simulink model "Counters"  (R2022a)
settings: Solver=FixedStepAuto  StartTime=0.0  StopTime=10.0  FixedStep=0.5  RelTol=1e-3
settings Model: Creator=SALAH  LastModifiedBy=SALAH

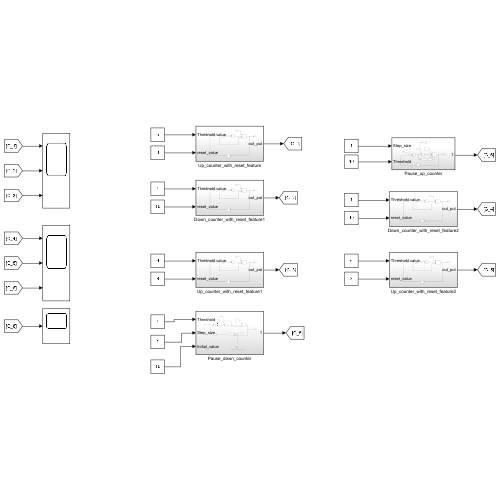
[thumbnail: Simulink's stored preview of the top-level diagram]
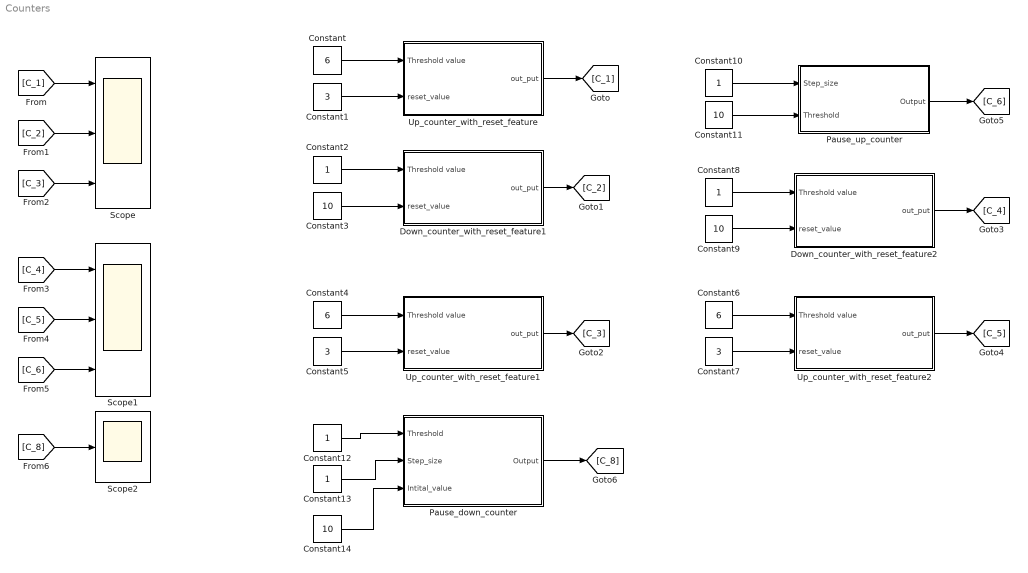
== system Counters ==
  Constant : Constant  Value=6
  Constant1 : Constant  Value=3
  Constant{2,8,10,12..13} (5 alike) : Constant
  Constant{3,9,11,14} (4 alike) : Constant  Value=10
  Constant4 : Constant  Value=6
  Constant5 : Constant  Value=3
  Constant6 : Constant  Value=6
  Constant7 : Constant  Value=3
  Down_counter_with_reset_feature1 : Subsystem
  Down_counter_with_reset_feature2 : Subsystem  Priority=2
  Pause_down_counter : Subsystem
  Pause_up_counter : Subsystem
  Scope : Scope  NumInputPorts=3
  Scope1 : Scope  NumInputPorts=3
  Scope2 : Scope
  Up_counter_with_reset_feature : Subsystem
  Up_counter_with_reset_feature1 : Subsystem
  Up_counter_with_reset_feature2 : Subsystem  Priority=1
  wires:
  Constant/1 -> Up_counter_with_reset_feature/1(Threshold value)
  Constant1/1 -> Up_counter_with_reset_feature/2(reset_value)
  Constant3/1 -> Down_counter_with_reset_feature1/2(reset_value)
  Constant2/1 -> Down_counter_with_reset_feature1/1(Threshold value)
  Constant5/1 -> Up_counter_with_reset_feature1/2(reset_value)
  Constant4/1 -> Up_counter_with_reset_feature1/1(Threshold value)
  Constant6/1 -> Up_counter_with_reset_feature2/1(Threshold value)
  Constant7/1 -> Up_counter_with_reset_feature2/2(reset_value)
  Up_counter_with_reset_feature/1(out_put) -> [C_1]
  Down_counter_with_reset_feature1/1(out_put) -> [C_2]
  Up_counter_with_reset_feature1/1(out_put) -> [C_3]
  Down_counter_with_reset_feature2/1(out_put) -> [C_4]
  Up_counter_with_reset_feature2/1(out_put) -> [C_5]
  [C_1] -> Scope/1
  [C_2] -> Scope/2
  [C_3] -> Scope/3
  [C_4] -> Scope1/1
  [C_5] -> Scope1/2
  Constant8/1 -> Down_counter_with_reset_feature2/1(Threshold value)
  Constant9/1 -> Down_counter_with_reset_feature2/2(reset_value)
  Constant10/1 -> Pause_up_counter/1(Step_size)
  Constant11/1 -> Pause_up_counter/2(Threshold)
  Pause_up_counter/1(Output) -> [C_6]
  [C_6] -> Scope1/3
  Constant12/1 -> Pause_down_counter/1(Threshold)
  Constant13/1 -> Pause_down_counter/2(Step_size)
  Pause_down_counter/1(Output) -> [C_8]
  [C_8] -> Scope2/1
  Constant14/1 -> Pause_down_counter/3(Intital_value)

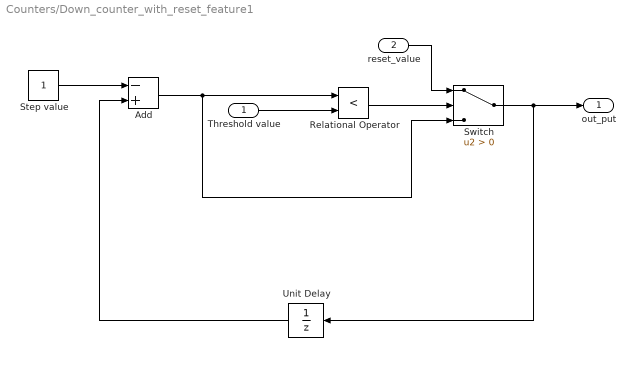
== system Counters/Down_counter_with_reset_feature1 ==
  Threshold value : Inport
  reset_value : Inport  Port=2
  Add : Sum  Inputs=-+
  Relational Operator : RelationalOperator  Operator=<  OutDataTypeStr=boolean  RndMeth=Simplest  InputSameDT=off
  Step value : Constant
  Switch : Switch  Criteria=u2 > Threshold  SaturateOnIntegerOverflow=off  InputSameDT=off
  Unit Delay : UnitDelay  SampleTime=-1  HasFrameUpgradeWarning=on
  out_put : Outport
  wires:
  reset_value/1 -> Switch/1
  Add/1 -> Relational Operator/1, Switch/3
  Unit Delay/1 -> Add/2
  Switch/1 -> Unit Delay/1, out_put/1
  Threshold value/1 -> Relational Operator/2
  Relational Operator/1 -> Switch/2
  Step value/1 -> Add/1

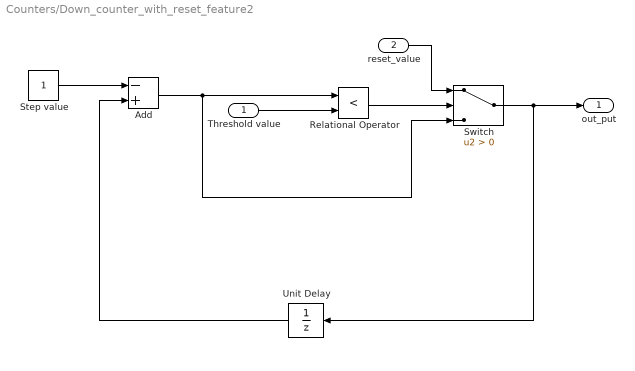
== system Counters/Down_counter_with_reset_feature2 ==
  Threshold value : Inport
  reset_value : Inport  Port=2
  Add : Sum  Inputs=-+
  Relational Operator : RelationalOperator  Operator=<  OutDataTypeStr=boolean  RndMeth=Simplest  InputSameDT=off
  Step value : Constant
  Switch : Switch  Criteria=u2 > Threshold  SaturateOnIntegerOverflow=off  InputSameDT=off
  Unit Delay : UnitDelay  SampleTime=-1  HasFrameUpgradeWarning=on
  out_put : Outport
  wires:
  Step value/1 -> Add/1
  Relational Operator/1 -> Switch/2
  Threshold value/1 -> Relational Operator/2
  Switch/1 -> out_put/1, Unit Delay/1
  Unit Delay/1 -> Add/2
  Add/1 -> Switch/3, Relational Operator/1
  reset_value/1 -> Switch/1

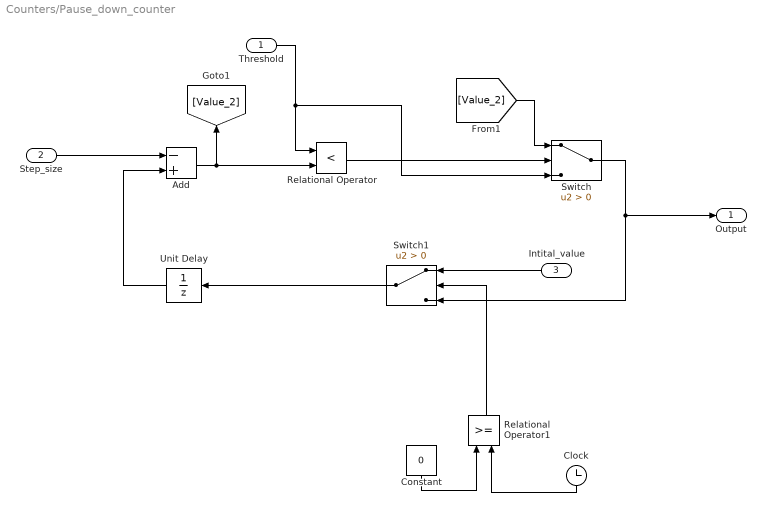
== system Counters/Pause_down_counter ==
  Threshold : Inport
  Step_size : Inport  Port=2
  Intital_value : Inport  Port=3
  Add : Sum  Inputs=-+
  Clock : Clock
  Constant : Constant  Value=0
  Relational Operator : RelationalOperator  Operator=<  OutDataTypeStr=boolean  RndMeth=Simplest  InputSameDT=off
  Relational Operator1 : RelationalOperator  Priority=1  OutDataTypeStr=boolean  RndMeth=Simplest  InputSameDT=off
  Switch : Switch  Criteria=u2 > Threshold  SaturateOnIntegerOverflow=off  InputSameDT=off
  Switch1 : Switch  Priority=2  Criteria=u2 > Threshold  SaturateOnIntegerOverflow=off  InputSameDT=off
  Unit Delay : UnitDelay  Priority=3  SampleTime=-1  HasFrameUpgradeWarning=on
  Output : Outport
  wires:
  Add/1 -> Relational Operator/2, [Value_2]
  Unit Delay/1 -> Add/2
  Relational Operator/1 -> Switch/2
  Threshold/1 -> Switch/3, Relational Operator/1
  Step_size/1 -> Add/1
  [Value_2] -> Switch/1
  Clock/1 -> Relational Operator1/2
  Constant/1 -> Relational Operator1/1
  Switch1/1 -> Unit Delay/1
  Switch/1 -> Switch1/3, Output/1
  Relational Operator1/1 -> Switch1/2
  Intital_value/1 -> Switch1/1

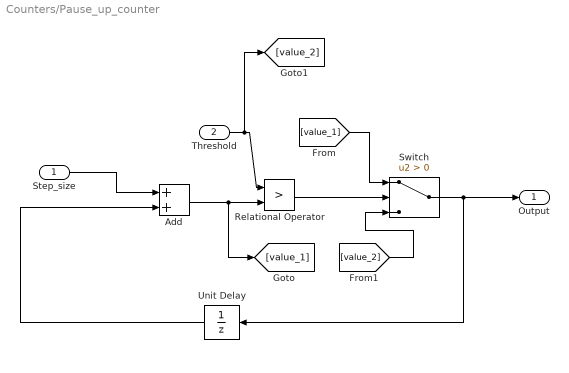
== system Counters/Pause_up_counter ==
  Step_size : Inport
  Threshold : Inport  Port=2
  Add : Sum
  Relational Operator : RelationalOperator  Operator=>  OutDataTypeStr=boolean  RndMeth=Simplest  InputSameDT=off
  Switch : Switch  Criteria=u2 > Threshold  SaturateOnIntegerOverflow=off  InputSameDT=off
  Unit Delay : UnitDelay  SampleTime=-1  HasFrameUpgradeWarning=on
  Output : Outport
  wires:
  Unit Delay/1 -> Add/2
  Step_size/1 -> Add/1
  Add/1 -> [value_1], Relational Operator/2
  Threshold/1 -> [value_2], Relational Operator/1
  Relational Operator/1 -> Switch/2
  Switch/1 -> Unit Delay/1, Output/1
  [value_1] -> Switch/1
  [value_2] -> Switch/3

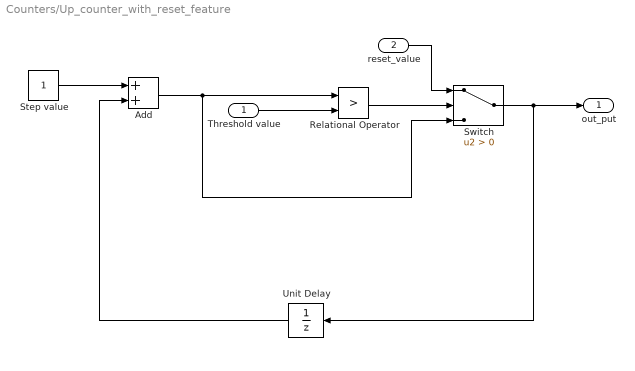
== system Counters/Up_counter_with_reset_feature ==
  Threshold value : Inport
  reset_value : Inport  Port=2
  Add : Sum
  Relational Operator : RelationalOperator  Operator=>  OutDataTypeStr=boolean  RndMeth=Simplest  InputSameDT=off
  Step value : Constant
  Switch : Switch  Criteria=u2 > Threshold  SaturateOnIntegerOverflow=off  InputSameDT=off
  Unit Delay : UnitDelay  SampleTime=-1  HasFrameUpgradeWarning=on
  out_put : Outport
  wires:
  Step value/1 -> Add/1
  Relational Operator/1 -> Switch/2
  Threshold value/1 -> Relational Operator/2
  Switch/1 -> out_put/1, Unit Delay/1
  Unit Delay/1 -> Add/2
  Add/1 -> Switch/3, Relational Operator/1
  reset_value/1 -> Switch/1

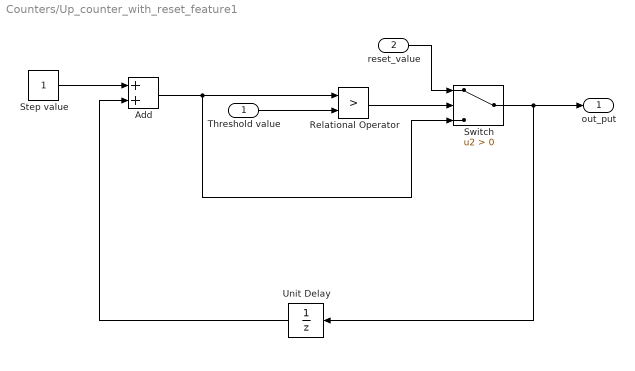
== system Counters/Up_counter_with_reset_feature1 ==
  Threshold value : Inport
  reset_value : Inport  Port=2
  Add : Sum
  Relational Operator : RelationalOperator  Operator=>  OutDataTypeStr=boolean  RndMeth=Simplest  InputSameDT=off
  Step value : Constant
  Switch : Switch  Criteria=u2 > Threshold  SaturateOnIntegerOverflow=off  InputSameDT=off
  Unit Delay : UnitDelay  SampleTime=-1  HasFrameUpgradeWarning=on
  out_put : Outport
  wires:
  reset_value/1 -> Switch/1
  Add/1 -> Relational Operator/1, Switch/3
  Unit Delay/1 -> Add/2
  Switch/1 -> Unit Delay/1, out_put/1
  Threshold value/1 -> Relational Operator/2
  Relational Operator/1 -> Switch/2
  Step value/1 -> Add/1

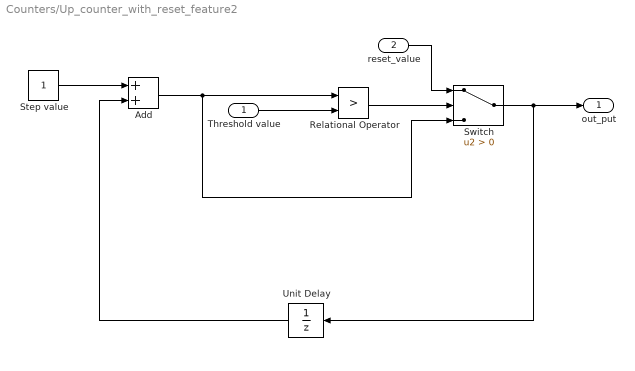
== system Counters/Up_counter_with_reset_feature2 ==
  Threshold value : Inport
  reset_value : Inport  Port=2
  Add : Sum
  Relational Operator : RelationalOperator  Operator=>  OutDataTypeStr=boolean  RndMeth=Simplest  InputSameDT=off
  Step value : Constant
  Switch : Switch  Criteria=u2 > Threshold  SaturateOnIntegerOverflow=off  InputSameDT=off
  Unit Delay : UnitDelay  SampleTime=-1  HasFrameUpgradeWarning=on
  out_put : Outport
  wires:
  Step value/1 -> Add/1
  Relational Operator/1 -> Switch/2
  Threshold value/1 -> Relational Operator/2
  Switch/1 -> out_put/1, Unit Delay/1
  Unit Delay/1 -> Add/2
  Add/1 -> Switch/3, Relational Operator/1
  reset_value/1 -> Switch/1
